simulink subsystem "Inputs_MotorDriveUnit_Random_refsub"  (R2026a)
settings: Solver=VariableStepAuto
libraries: simulink x1
settings Model: Creator=isaacito  LastModifiedBy=isaacito

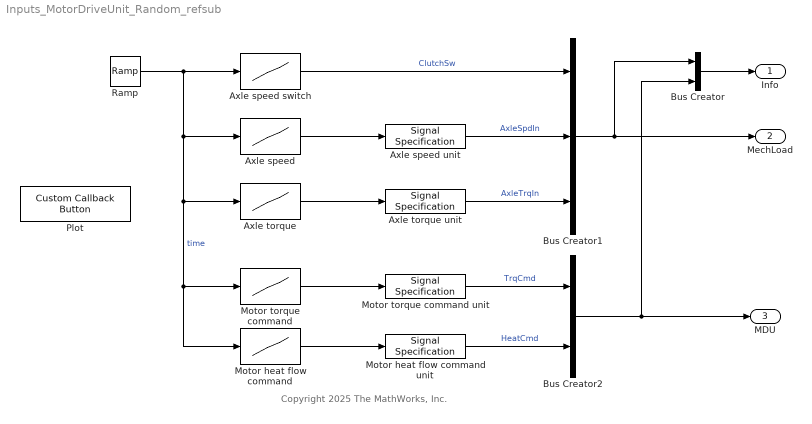
== system Inputs_MotorDriveUnit_Random_refsub ==
  note: Copyright 2025 The MathWorks, Inc.
  Axle speed : Lookup_n-D  NumberOfTableDimensions=1  BreakpointsForDimension1=[0; 50; 100]  Table=[0; 0; 0]  InterpMethod=Akima spline  InternalRulePriority=Speed  RndMeth=Simplest
  Axle speed switch : Lookup_n-D  NumberOfTableDimensions=1  BreakpointsForDimension1=[0, 1]  Table=[0, 0]  InterpMethod=Flat  InternalRulePriority=Speed  RndMeth=Simplest
  Axle speed unit : SignalSpecification  Unit=rpm
  Axle torque : Lookup_n-D  NumberOfTableDimensions=1  BreakpointsForDimension1=[0; 2.5; 5; 10; 12.5; 15; 16; 17; 18; 19; 20.5; 22; 23; 23.5; 24; 25; 26.5; 28; 31; 32.5; 34; 37; 39.5; 42; 43; 45.5; 48; 50; 51; 52; 55; 57; 59; 60; 61; 62; 65; 66; 67; 68; 70.5; 73; 75; 76.5; 78; 79; 79.5; 80; 83; 84.5; 86; 89; 89.5; 90; 91; 93.5; 96; 99; 100.5; 102; 104; 105.5; 107; 109; 109.5; 110; 112; 113; 114; 115; 117.5; 120; 122; 122.5; 123; 126; 128.5; 131; 132; 132.5; 133; 135; 135.5; 136; 138; 140; 142; 144; 144.5; 145; 147; 148.5; 150; 153; 153.5; 154; 157; 158.5; 160; 162; 164; 166; 169; 169.5; 170; 172; 174; 176; 178; 179; 180; 181; 183; 185; 187; 188.5; 190; 192; 194; 196; 197; 198.5; 200; 201; 203.5; 206; 209; 211; 213; 216; 217; 218; 220; 221.5; 223; 226; 227; 228; 231; 231.5; 232; 234; 235.5; 237; 238; 239.5; 241; 243; 245.5; 248; 251; 252; 253; 256; 258.5; 261; 262; 263; 264; 267; 268; 269; 270; 272; 274; 276; 277.5; 279; 281; 282; 283; 285; 287.5; 290; 293; 293.5; 294; 296; 297; 298; 300; 302; 304; 305; 307; 309; 311; 316; 321]  Table=[0; 0; 0; -8; -8; -8; -8; -8; -8; -6; -6; -6; -6; -6; -6; -9; -9; -9; -10; -10; -10; -3; -3; -3; -8; -8; -8; -6; -6; -6; -4; -4; -4; -8; -8; -8; -5; -5; -5; -6; -6; -6; -3; -3; -3; -5; -5; -5; -6; -6; -6; -5; -5; -5; -7; -7; -7; -7; -7; -7; -3; -3; -3; -10; -10; -10; -6; -6; -6; -8; -8; -8; -7; -7; -7; -8; -8; -8; -4; -4; -4; -10; -10; -10; -3; -3; -3; -10; -10; -10; -8; -8; -8; -10; -10; -10; -10; -10; -10; -9; -9; -9; -9; -9; -9; -9; -9; -9; -3; -3; -3; -7; -7; -7; -4; -4; -4; -3; -3; -3; -4; -4; -4; -6; -6; -6; -3; -3; -3; -8; -8; -8; -8; -8; -8; -9; -9; -9; -4; -4; -4; -10; -10; -10; -7; -7; -7; -4; -4; -4; -10; -10; -10; -5; -5; -5; -8; -8; -8; -8; -8; -8; -5; -5; -5; -7; -7; -7; -8; -8; -8; -9; -9; -9; -6; -6; -6; -7; -7; -7; -3; -3; -3; -5; -5; -5; 0; 0; 0]  InterpMethod=Akima spline  InternalRulePriority=Speed  RndMeth=Simplest
  Axle torque unit : SignalSpecification  Unit=N*m
  Bus Creator : BusCreator  Inputs=2
  Bus Creator1 : BusCreator  Inputs=3
  Bus Creator2 : BusCreator  Inputs=2
  Motor heat flow command : Lookup_n-D  NumberOfTableDimensions=1  BreakpointsForDimension1=[0; 50; 100]  Table=[0; 0; 0]  InterpMethod=Akima spline  InternalRulePriority=Speed  RndMeth=Simplest
  Motor heat flow command unit : SignalSpecification  Unit=W
  Motor torque command : Lookup_n-D  NumberOfTableDimensions=1  BreakpointsForDimension1=[0; 2.5; 5; 10; 15; 20; 22; 26; 30; 32; 39; 46; 48; 57; 66; 68; 70; 72; 76; 82.5; 89; 94; 101; 108; 111; 117; 123; 126; 132; 138; 143; 150.5; 158; 160; 167.5; 175; 180; 184.5; 189; 191; 198.5; 206; 209; 215.5; 222; 224; 230; 236; 241; 245; 249; 254; 259; 264; 266; 271.5; 277; 282; 286; 290; 293; 297; 301; 305; 313; 321; 323; 328; 333]  Table=[0; 0; 0; 69; 69; 69; 45; 45; 45; 84; 84; 84; 73; 73; 73; 51; 51; 51; 23; 23; 23; 35; 35; 35; 90; 90; 90; 88; 88; 88; 22; 22; 22; 98; 98; 98; 15; 15; 15; 36; 36; 36; 40; 40; 40; 63; 63; 63; 100; 100; 100; 57; 57; 57; 58; 58; 58; 0; 0; 0; 85; 85; 85; 21; 21; 21; 0; 0; 0]  InterpMethod=Akima spline  InternalRulePriority=Speed  RndMeth=Simplest
  Motor torque command unit : SignalSpecification  Unit=N*m
  Plot : CustomCallbackButton  Configuration="{\"components\":[{\"name\":\"BackgroundImageComponent\",\"settings\":{\"image\":{\"size\":[0,0],\"src\":\"default\",\"srcOrientation\":\"Right\"},\"position\":[0,0,1,1]}},{\"name\":\"ButtonStateComponent\",\"settings\":{\"buttonType\":\"momentary\",\"clickFcn\":\"% Specify blocks to sort plot order.\\nblocks = [\\n  \\\"Axle speed switch\\\"\\n  \\\"Axle speed\\\"\\n  \\\"Axle torque\\\"\\n  \\\"Motor torque command\\\"\\n  \\\"Motor heat flow command\\\"\\n];\\nbevutil1.ModelUtil.plotLookupTable1DBlocks(gcs, Blocks=blocks, DivisionType=\\\"InterpolationInterval\\\", InterpolationInterval=0.1)\",\"onValue\":1,\"position\":[0,0,1,1],\"pressDelay\":\"500\",\"pressFcn\":\"\",\"repeatInterval\":\"0\",\"states\":[{\"horizontalAlignment\":\"center\",\"image\":{\"position\":[0,0,1,1],\"size\":[1,1],\"src\":\"default\",\"srcOrientation\":\"Right\"},\"label\":{\"color\":[0.01176470588,0.01176470588,0.01176470588,1],\"icon\":{\"size\":[0,0],\"src\":\"default\",\"srcOrientation\":\"Right\"},\"iconOffset\":0,\"iconPlacement\":\"left\",\"opacity\":1,\"show\":true,\"text\":{\"content\":\"Lookup tables\",\"font\":\"Helvetica\"}},\"labelOffset\":[0,0],\"verticalAlignment\":\"middle\"},{\"horizontalAlignment\":\"center\",\"image\":{\"position\":[0,0,1,1],\"size\":[1,1],\"src\":\"default\",\"srcOrientation\":\"Right\"},\"label\":{\"color\":[0.01176470588,0.01176470588,0.01176470588,1],\"icon\":{\"size\":[0,0],\"src\":\"default\",\"srcOrientation\":\"Right\"},\"iconOffset\":0,\"iconPlacement\":\"left\",\"opacity\":1,\"show\":true,\"text\":{\"content\":\"Lookup tables\",\"font\":\"Helvetica\"}},\"labelOffset\":[0,0],\"verticalAlignment\":\"middle\"},{\"horizontalAlignment\":\"center\",\"image\":{\"position\":[0,0,1,1],\"size\":[1,1],\"src\":\"default\",\"srcOrientation\":\"Right\"},\"label\":{\"color\":[0.01176470588,0.01176470588,0.01176470588,1],\"icon\":{\"size\":[0,0],\"src\":\"default\",\"srcOrientation\":\"Right\"},\"iconOffset\":0,\"iconPlacement\":\"left\",\"opacity\":1,\"show\":true,\"text\":{\"content\":\"Lookup tables\",\"font\":\"Helvetica\"}},\"labelOffset\":[0,0],\"verticalAlignment\":\"middle\"},{\"horizontalAlignment\":\"center\",\"image\":{\"position\":[0,0,1,1],\"size\":[1,1],\"src\":\"default\",\"srcOrientation\":\"Right\"},\"label\":{\"color\":[0.01176470588,0.01176470588,0.01176470588,1],\"icon\":{\"size\":[0,0],\"src\":\"default\",\"srcOrientation\":\"Right\"},\"iconOffset\":0,\"iconPlacement\":\"left\",\"opacity\":1,\"show\":true,\"text\":{\"content\":\"Lookup tables\",\"font\":\"Helvetica\"}},\"labelOffset\":[0,0],\"verticalAlignment\":\"middle\"}]}},{\"name\":\"ForegroundImageComponent\",\"settings\":{\"image\":{\"size\":[0,0],\"src\":\"default\",\"srcOrientation\":\"Right\"},\"isForeground\":1,\"position\":[0,0,1,1]}}],\"derived\":{\"blockParameters\":{\"AutoActivate\":true,\"ButtonText\":\"Lookup tables\",\"ButtonType\":\"Momentary\",\"ClickFcn\":\"% Specify blocks to sort plot order.\\nblocks = [\\n  \\\"Axle speed switch\\\"\\n  \\\"Axle speed\\\"\\n  \\\"Axle torque\\\"\\n  \\\"Motor torque command\\\"\\n  \\\"Motor heat flow command\\\"\\n];\\nbevutil1.ModelUtil.plotLookupTable1DBlocks(gcs, Blocks=blocks, DivisionType=\\\"InterpolationInterval\\\", InterpolationInterval=0.1)\",\"OnValue\":1,\"PressDelay\":\"500\",\"PressFcn\":\"\",\"RepeatInterval\":\"0\",\"fixedAspectRatio\":\"off\"}},\"settings\":{\"BindingType\":\"standalone\",\"autoActivate\":true,\"backgroundColor\":[244,244,244,1],\"backgroundOffset\":0.2,\"backgroundOpacity\":1,\"fixedAspectRatio\":\"off\",\"foregroundColor\":[0.01176470588,0.01176470588,0.01176470588,1],\"migratedFromLegacy\":true,\"useBackgroundColor\":true,\"variant\":\"callback\",\"version\":\"R2025a\"},\"type\":\"Button\"}"  CustomBackgroundColor="{\"color\":[0.9568627451,0.9568627451,0.9568627451],\"show\":true}"
  Ramp : simulink/Sources/Ramp  slope=1  start=0  InitialOutput=0
      settings: AttributesFormatString=|
      | Slope: %<slope>
      | Start time: %<start>
      | Initial output: %<InitialOutput>
  Info : Outport
  MechLoad : Outport  Port=2
  MDU : Outport  Port=3
  wires:
  Bus Creator/1 -> Info/1
  Motor torque command unit/1 -> Bus Creator2/1  "TrqCmd"
  Axle torque unit/1 -> Bus Creator1/3  "AxleTrqIn"
  Axle speed unit/1 -> Bus Creator1/2  "AxleSpdIn"
  Motor heat flow command unit/1 -> Bus Creator2/2  "HeatCmd"
  Bus Creator2/1 -> Bus Creator/2, MDU/1
  Bus Creator1/1 -> Bus Creator/1, MechLoad/1
  Ramp/1 -> Motor heat flow command/1, Motor torque command/1, Axle torque/1, Axle speed/1, Axle speed switch/1  "time"
  Axle speed switch/1 -> Bus Creator1/1  "ClutchSw"
  Axle speed/1 -> Axle speed unit/1
  Axle torque/1 -> Axle torque unit/1
  Motor torque command/1 -> Motor torque command unit/1
  Motor heat flow command/1 -> Motor heat flow command unit/1
